simulink model "openloop"  (R2023a)
settings: Solver=VariableStepAuto  StartTime=0.0  StopTime=4  RelTol=1e-3
libraries: spsSeriesRLCBranchLib x4, spsACVoltageSourceLib x3, spsUniversalBridgeLib x2, spsDCMachineLib x1, spsDCVoltageSourceLib x1, spsMeanLib x1, spsVoltageMeasurementLib x1, sps_lib x1
settings Model: Creator=User  LastModifiedBy=User
settings SolverCC: ZeroCrossControl=EnableAll
settings DebuggingCC: IgnoredZcDiagnostic=none

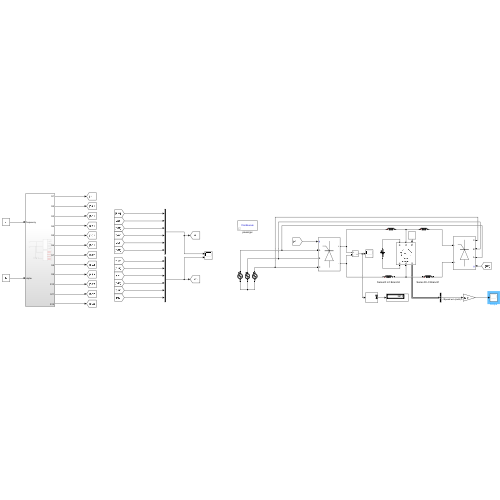
[thumbnail: Simulink's stored preview of the top-level diagram]
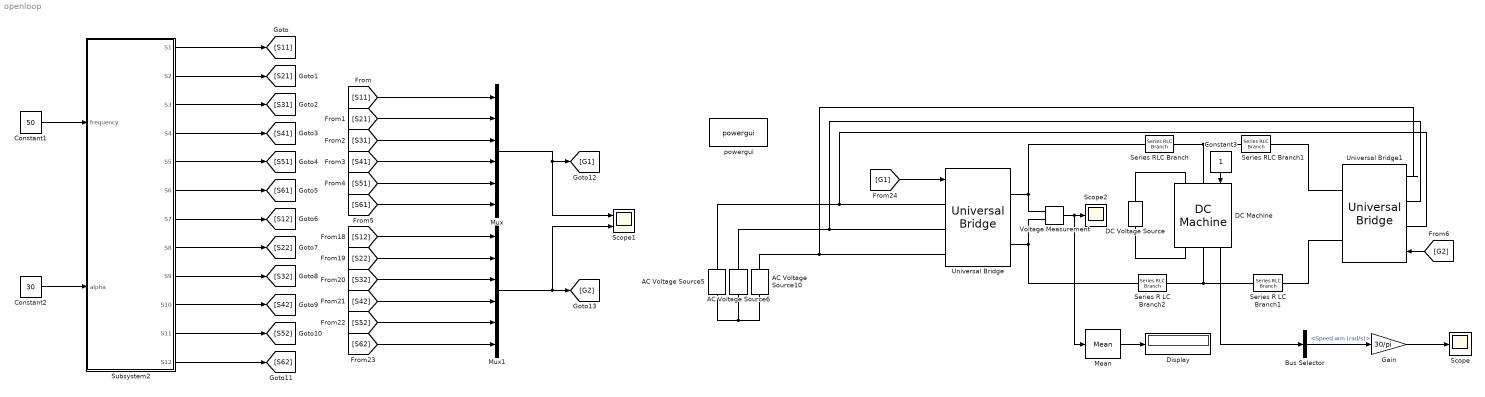
== system openloop ==
  AC Voltage Source10 : spsACVoltageSourceLib/AC Voltage Source  Amplitude=220  Phase=120  Frequency=50  SampleTime=0  Measurements=None  BusType=swing  Pref=10e3  Qref=0  Qmin=-inf  Qmax=+inf
  AC Voltage Source5 : spsACVoltageSourceLib/AC Voltage Source  Amplitude=220  Phase=0  Frequency=50  SampleTime=0  Measurements=None  BusType=swing  Pref=10e3  Qref=0  Qmin=-inf  Qmax=+inf
  AC Voltage Source6 : spsACVoltageSourceLib/AC Voltage Source  Amplitude=220  Phase=-120  Frequency=50  SampleTime=0  Measurements=None  BusType=swing  Pref=10e3  Qref=0  Qmin=-inf  Qmax=+inf
  Bus Selector : BusSelector  OutputSignals=Speed wm (rad/s)
  Constant1 : Constant  Value=50
  Constant2 : Constant  Value=30
  Constant3 : Constant
  DC Machine : spsDCMachineLib/DC Machine  PresetModel=03: 5HP 500V 1750RPM Field:300V  MechanicalLoad=Torque TL  FieldType=Wound  ShowDetailedParameters=on  MeasurementBus=off  RLa=[11.2 0.1215]  RLf=[281.2 156]  Laf=1.976  MachineConstant=Torque constant (N.m/A)  Ke=1.8  Kt=1.8  J=0.02215  Bm=0.002953  Tf=0.5161  w0=1  Ifinit=1.06685633001422  TsPowergui=0  TsBlock=-1
  DC Voltage Source : spsDCVoltageSourceLib/DC Voltage Source  Amplitude=300  Measurements=None
  Display : Display
  Gain : Gain  Gain=30/pi
  Mean : spsMeanLib/Mean  Freq=60  Vinit=0  Ts=0
  Mux : Mux  Inputs=6
  Mux1 : Mux  Inputs=6
  Scope : Scope
  Scope1 : Scope  NumInputPorts=2
  Scope2 : Scope
  Series R LC Branch1 : spsSeriesRLCBranchLib/Series RLC Branch  LConnTagsString=__new0  RConnTagsString=__new0  BranchType=L  Resistance=1  Inductance=0.083333333333333329  SetiL0=off  InitialCurrent=0  Capacitance=1e-6  Setx0=off  InitialVoltage=0  Measurements=None
  Series R LC Branch2 : spsSeriesRLCBranchLib/Series RLC Branch  LConnTagsString=__new0  RConnTagsString=__new0  BranchType=L  Resistance=1  Inductance=0.083333333333333329  SetiL0=off  InitialCurrent=0  Capacitance=1e-6  Setx0=off  InitialVoltage=0  Measurements=None
  Series RLC Branch : spsSeriesRLCBranchLib/Series RLC Branch  LConnTagsString=__new0  RConnTagsString=__new0  BranchType=L  Resistance=1  Inductance=0.083333333333333329  SetiL0=off  InitialCurrent=0  Capacitance=1e-6  Setx0=off  InitialVoltage=0  Measurements=None
  Series RLC Branch1 : spsSeriesRLCBranchLib/Series RLC Branch  LConnTagsString=__new0  RConnTagsString=__new0  BranchType=L  Resistance=1  Inductance=0.083333333333333329  SetiL0=off  InitialCurrent=0  Capacitance=1e-6  Setx0=off  InitialVoltage=0  Measurements=None
  Subsystem2 : Subsystem
  Universal Bridge : spsUniversalBridgeLib/Universal Bridge  Arms=3  SnubberResistance=1e5  SnubberCapacitance=inf  Device=Thyristors  Ron=1e-3  Lon=0  ForwardVoltages="[  0  0  ]"  ForwardVoltage=0  GTOparameters=[ 10e-6 , 20e-6 ]  IGBTparameters=[ 1e-6 , 2e-6 ]  Measurements=None  Measurements_2=None  converterType=Rectifier
  Universal Bridge1 : spsUniversalBridgeLib/Universal Bridge  Arms=3  SnubberResistance=1e5  SnubberCapacitance=inf  Device=Thyristors  Ron=1e-3  Lon=0  ForwardVoltages="[  0  0  ]"  ForwardVoltage=0  GTOparameters=[ 10e-6 , 20e-6 ]  IGBTparameters=[ 1e-6 , 2e-6 ]  Measurements=None  Measurements_2=None  converterType=Rectifier
  Voltage Measurement : spsVoltageMeasurementLib/Voltage Measurement  PhasorSimulation=off  OutputType=Complex  PSBequivalent=0
  powergui : sps_lib/powergui  Priority=1  SimulationMode=Continuous  SampleTime=1e-6  frequency=60  Iterations=50  frequencyindice=0  Pbase=100e6  ErrMax=1e-4  UnitsV=kV  UnitsW=MW  buscounter=0  FunctionMessages=off  echomessages=off  EnableUseOfTLC=off  CurrentSourceSwitches=off  DisableSnubberDevices=on  DisableRonSwitches=off  DisableVfSwitches=off  DisplayEquations=off  AutomaticDiscreteSolvers=off  SolverType=Tustin/Backward Euler (TBE)  Interpol=off  ExternalGateDelay=off  methode=off  Ts=100  x0status=blocks  SPID=on  SwTol=0  HookPort=off  NonlinearTolerance=1e-4  nMaxIteration=100  ContinueOnMaxIteration=off  RestoreLinks=warning  ResistiveCurrentMeasurement=off  Frange=[0:2:500]  Ylog=off  Xlog=on  ShowGrid=off  save=off  variable=ZData  structure=0  ZoomFFT=off  StartTime=0.0  cycles=1  DisplayStyle=1  fundamental=60  FreqAxis=off  MaxFrequency=1000  frequencyindicesteady=1  RmsSteady=1  display=off
  wires:
  DC Machine/1 -> Bus Selector/1
  Bus Selector/1 -> Gain/1  "<Speed wm (rad/s)>"
  Gain/1 -> Scope/1
  [S11] -> Mux/1
  [S21] -> Mux/2
  [S31] -> Mux/3
  [S41] -> Mux/4
  [S51] -> Mux/5
  [S61] -> Mux/6
  Constant3/1 -> DC Machine/1
  Constant1/1 -> Subsystem2/1(frequency)
  Constant2/1 -> Subsystem2/2(alpha)
  Subsystem2/1(S1) -> [S11]
  Subsystem2/2(S2) -> [S21]
  Subsystem2/3(S3) -> [S31]
  Subsystem2/4(S4) -> [S41]
  Subsystem2/5(S5) -> [S51]
  Subsystem2/6(S6) -> [S61]
  Subsystem2/7(S7) -> [S12]
  Subsystem2/8(S8) -> [S22]
  Subsystem2/9(S9) -> [S32]
  Subsystem2/10(S10) -> [S42]
  Subsystem2/11(S11) -> [S52]
  Subsystem2/12(S12) -> [S62]
  Voltage Measurement/1 -> Mean/1, Scope2/1
  Mean/1 -> Display/1
  [S62] -> Mux1/6
  [S52] -> Mux1/5
  [S42] -> Mux1/4
  [S32] -> Mux1/3
  [S22] -> Mux1/2
  [S12] -> Mux1/1
  Mux/1 -> [G1], Scope1/1
  Mux1/1 -> Scope1/2, [G2]
  [G1] -> Universal Bridge/1
  [G2] -> Universal Bridge1/1
  connections:
  Voltage Measurement/LConn2 -- Universal Bridge/RConn2 -- Series R LC Branch2/LConn1
  DC Voltage Source/RConn1 -- DC Machine/LConn2
  DC Voltage Source/LConn1 -- DC Machine/RConn2
  AC Voltage Source10/LConn1 -- AC Voltage Source6/LConn1 -- AC Voltage Source5/LConn1
  Voltage Measurement/LConn1 -- Universal Bridge/RConn1 -- Series RLC Branch/LConn1
  Series RLC Branch/RConn1 -- Series RLC Branch1/LConn1 -- DC Machine/LConn1
  Series R LC Branch1/LConn1 -- Series R LC Branch2/RConn1 -- DC Machine/RConn1
  Universal Bridge/LConn1 -- Universal Bridge1/LConn1 -- AC Voltage Source5/RConn1
  AC Voltage Source6/RConn1 -- Universal Bridge1/LConn2 -- Universal Bridge/LConn2
  Universal Bridge/LConn3 -- Universal Bridge1/LConn3 -- AC Voltage Source10/RConn1
  Universal Bridge1/RConn2 -- Series RLC Branch1/RConn1
  Universal Bridge1/RConn1 -- Series R LC Branch1/RConn1

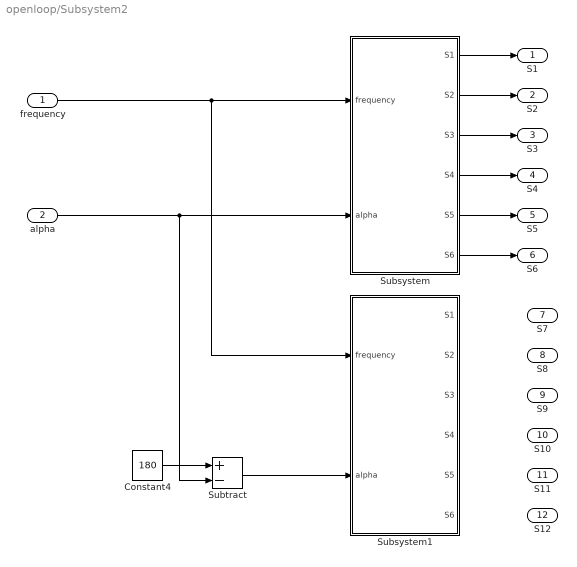
== system openloop/Subsystem2 ==
  frequency : Inport
  alpha : Inport  Port=2
  Constant4 : Constant  Value=180
  Subsystem : Subsystem
  Subsystem1 : Subsystem
  Subtract : Sum  Inputs=+-
  S1 : Outport
  S2 : Outport  Port=2
  S3 : Outport  Port=3
  S4 : Outport  Port=4
  S5 : Outport  Port=5
  S6 : Outport  Port=6
  S7 : Outport  Port=7
  S8 : Outport  Port=8
  S9 : Outport  Port=9
  S10 : Outport  Port=10
  S11 : Outport  Port=11
  S12 : Outport  Port=12
  wires:
  Constant4/1 -> Subtract/1
  frequency/1 -> Subsystem1/1(frequency), Subsystem/1(frequency)
  Subtract/1 -> Subsystem1/2(alpha)
  Subsystem/3(S3) -> S3/1
  Subsystem/2(S2) -> S2/1
  ? -> S11/1
  Subsystem/1(S1) -> S1/1
  ? -> S10/1
  alpha/1 -> Subtract/2, Subsystem/2(alpha)
  ? -> S9/1
  Subsystem/6(S6) -> S6/1
  Subsystem/4(S4) -> S4/1
  Subsystem/5(S5) -> S5/1
  ? -> S8/1
  ? -> S7/1
  ? -> S12/1

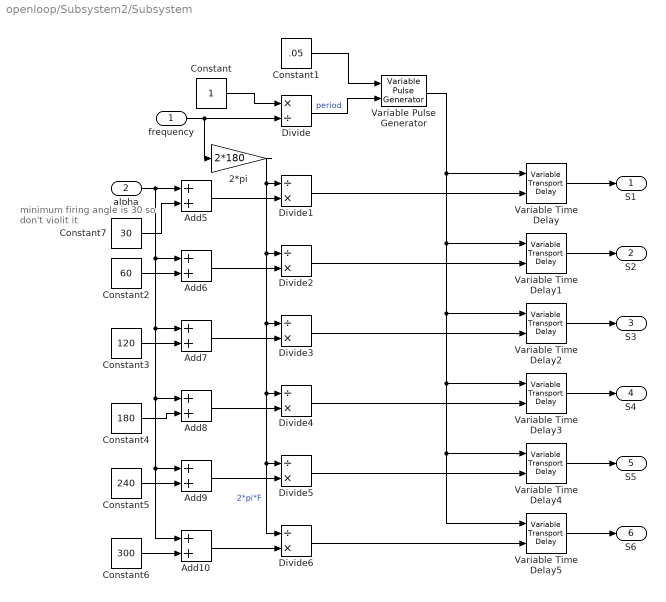
== system openloop/Subsystem2/Subsystem ==
  note: minimum firing angle is 30 so don't violit it
  frequency : Inport
  alpha : Inport  Port=2
  2*pi : Gain  Gain=2*180
  Add{5..10} (6 alike) : Sum
  Constant : Constant
  Constant1 : Constant  Value=.05
  Constant2 : Constant  Value=60
  Constant3 : Constant  Value=120
  Constant4 : Constant  Value=180
  Constant5 : Constant  Value=240
  Constant6 : Constant  Value=300
  Constant7 : Constant  Value=30
  Divide : Product  Inputs=*/
  Divide{1..6} (6 alike) : Product  Inputs=/*
  Variable Time Delay{,1..5} (6 alike) : VariableTransportDelay  MaximumDelay=10
  Variable Pulse Generator : VariablePulseGenerator  SampleTime=0.1
  S1 : Outport
  S2 : Outport  Port=2
  S3 : Outport  Port=3
  S4 : Outport  Port=4
  S5 : Outport  Port=5
  S6 : Outport  Port=6
  wires:
  frequency/1 -> 2*pi/1, Divide/2
  Constant/1 -> Divide/1
  Divide/1 -> Variable Pulse Generator/2  "period"
  Constant1/1 -> Variable Pulse Generator/1
  Variable Pulse Generator/1 -> Variable Time Delay2/1, Variable Time Delay4/1, Variable Time Delay5/1, Variable Time Delay3/1, Variable Time Delay1/1, Variable Time Delay/1
  Variable Time Delay/1 -> S1/1
  Variable Time Delay1/1 -> S2/1
  Variable Time Delay2/1 -> S3/1
  Variable Time Delay4/1 -> S5/1
  Variable Time Delay3/1 -> S4/1
  Variable Time Delay5/1 -> S6/1
  alpha/1 -> Add10/1, Add9/1, Add8/1, Add7/1, Add6/1, Add5/1
  2*pi/1 -> Divide6/1, Divide5/1, Divide4/1, Divide3/1, Divide2/1, Divide1/1  "2*pi*F"
  Divide1/1 -> Variable Time Delay/2
  Divide2/1 -> Variable Time Delay1/2
  Divide3/1 -> Variable Time Delay2/2
  Divide4/1 -> Variable Time Delay3/2
  Divide5/1 -> Variable Time Delay4/2
  Divide6/1 -> Variable Time Delay5/2
  Constant2/1 -> Add6/2
  Constant3/1 -> Add7/2
  Constant4/1 -> Add8/2
  Constant5/1 -> Add9/2
  Constant6/1 -> Add10/2
  Add5/1 -> Divide1/2
  Constant7/1 -> Add5/2
  Add6/1 -> Divide2/2
  Add7/1 -> Divide3/2
  Add8/1 -> Divide4/2
  Add9/1 -> Divide5/2
  Add10/1 -> Divide6/2

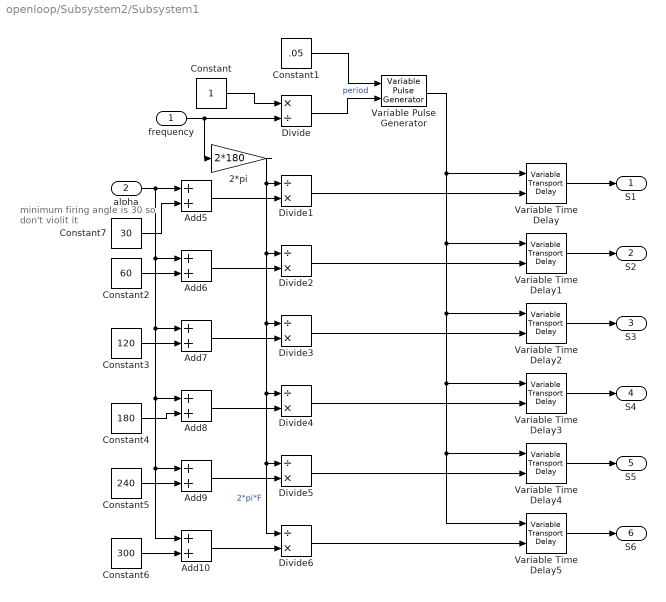
== system openloop/Subsystem2/Subsystem1 ==
  note: minimum firing angle is 30 so don't violit it
  frequency : Inport
  alpha : Inport  Port=2
  2*pi : Gain  Gain=2*180
  Add{5..10} (6 alike) : Sum
  Constant : Constant
  Constant1 : Constant  Value=.05
  Constant2 : Constant  Value=60
  Constant3 : Constant  Value=120
  Constant4 : Constant  Value=180
  Constant5 : Constant  Value=240
  Constant6 : Constant  Value=300
  Constant7 : Constant  Value=30
  Divide : Product  Inputs=*/
  Divide{1..6} (6 alike) : Product  Inputs=/*
  Variable Time Delay{,1..5} (6 alike) : VariableTransportDelay  MaximumDelay=10
  Variable Pulse Generator : VariablePulseGenerator  SampleTime=0.1
  S1 : Outport
  S2 : Outport  Port=2
  S3 : Outport  Port=3
  S4 : Outport  Port=4
  S5 : Outport  Port=5
  S6 : Outport  Port=6
  wires:
  Divide3/1 -> Variable Time Delay2/2
  Add7/1 -> Divide3/2
  Variable Time Delay4/1 -> S5/1
  Constant2/1 -> Add6/2
  Add8/1 -> Divide4/2
  Add9/1 -> Divide5/2
  Add10/1 -> Divide6/2
  Divide2/1 -> Variable Time Delay1/2
  alpha/1 -> Add10/1, Add9/1, Add8/1, Add7/1, Add6/1, Add5/1
  Constant3/1 -> Add7/2
  Constant7/1 -> Add5/2
  Add5/1 -> Divide1/2
  Add6/1 -> Divide2/2
  2*pi/1 -> Divide6/1, Divide5/1, Divide4/1, Divide3/1, Divide2/1, Divide1/1  "2*pi*F"
  Variable Time Delay1/1 -> S2/1
  Constant6/1 -> Add10/2
  Variable Time Delay/1 -> S1/1
  Divide4/1 -> Variable Time Delay3/2
  frequency/1 -> 2*pi/1, Divide/2
  Variable Time Delay2/1 -> S3/1
  Divide5/1 -> Variable Time Delay4/2
  Variable Pulse Generator/1 -> Variable Time Delay2/1, Variable Time Delay4/1, Variable Time Delay5/1, Variable Time Delay3/1, Variable Time Delay1/1, Variable Time Delay/1
  Divide1/1 -> Variable Time Delay/2
  Divide6/1 -> Variable Time Delay5/2
  Divide/1 -> Variable Pulse Generator/2  "period"
  Constant1/1 -> Variable Pulse Generator/1
  Variable Time Delay3/1 -> S4/1
  Variable Time Delay5/1 -> S6/1
  Constant/1 -> Divide/1
  Constant4/1 -> Add8/2
  Constant5/1 -> Add9/2
